simulink model "Hexacopter_2"  (R2017b)
settings: Solver=FixedStepAuto  StartTime=0.0  StopTime=50  FixedStep=0.0001  RelTol=1e-3
values from neighbouring files (symbols this model uses):
  b = 1.14 * 10^(-7)    (= 1.14e-07)    [hexa_parameters.m]
  dPhi_d = 0.0    (= 0)    [hexa_parameters.m]
  dPsi_d = 0.0    (= 0)    [hexa_parameters.m]
  dTheta_d = 0.0    (= 0)    [hexa_parameters.m]
  dx_0 = 0.0    (= 0)    [hexa_parameters.m]
  dy_0 = 0.0    (= 0)    [hexa_parameters.m]
  dz_0 = 0.0    (= 0)    [hexa_parameters.m]
  g = 9.81    [hexa_parameters.m]
  Ir = 3.36 * 10^(-5)    (= 3.36e-05)    [hexa_parameters.m]
  Ixx = 8.80 * 10^(-3)    (= 0.0088)    [hexa_parameters.m]
  Iyy = Ixx    (= 0.0088)    [hexa_parameters.m]
  Izz = 8.80 * 10^(-3)    (= 0.0088)    [hexa_parameters.m]
  k = 2.98 * 10^(-6)    (= 2.98e-06)    [hexa_parameters.m]
  Kphi_d = 0.01    [hexa_parameters.m]
  Kphi_p = 0.01    [hexa_parameters.m]
  Kpsi_d = 0.01    [hexa_parameters.m]
  Kpsi_p = 0.01    [hexa_parameters.m]
  Ktheta_d = 0.01    [hexa_parameters.m]
  Ktheta_p = 0.01    [hexa_parameters.m]
  Kz = 0.1    [hexa_parameters.m]
  Kzd = 1    [hexa_parameters.m]
  l = 1.0    (= 1)    [hexa_parameters.m]
  m = 0.468    [hexa_parameters.m]
  omega = 0.33    [hexa_parameters.m]
  p0 = 0.0    (= 0)    [hexa_parameters.m]
  Phi_d = 0.0    (= 0)    [hexa_parameters.m]
  Psi_d = 0.0    (= 0)    [hexa_parameters.m]
  q0 = 0.0    (= 0)    [hexa_parameters.m]
  q_0 = normalizer_quater(q_0)    [hexa_parameters.m]
  r0 = 0.0    (= 0)    [hexa_parameters.m]
  Theta_d = 0.0    (= 0)    [hexa_parameters.m]
  x_0 = 0.0    (= 0)    [hexa_parameters.m]
  y_0 = 0.0    (= 0)    [hexa_parameters.m]
  z_0 = 1.0    (= 1)    [hexa_parameters.m]
settings Model: Creator=Marco  LastModifiedBy=Marco
settings CodeAppCC: StateflowObjectComments=on

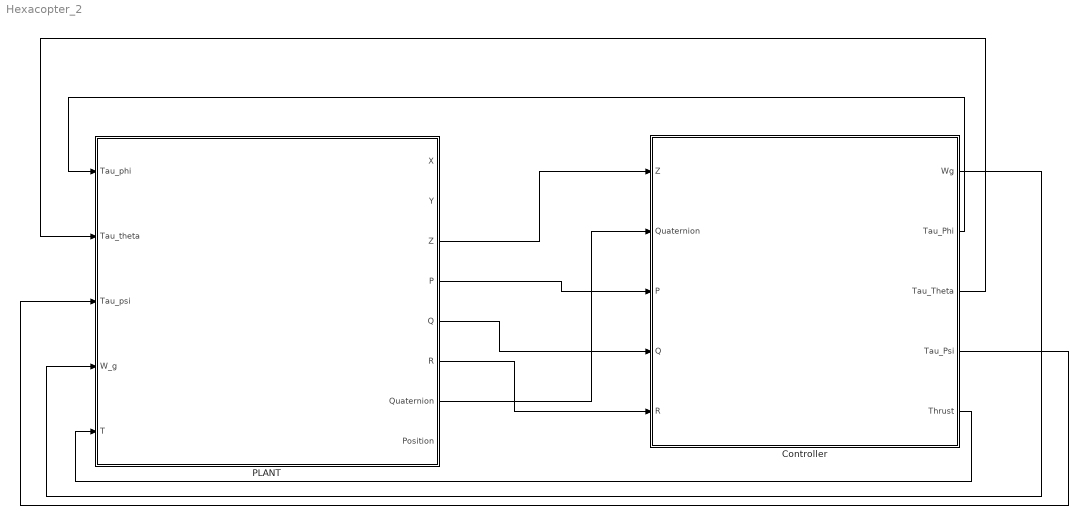
== system Hexacopter_2 ==
  Controller : Subsystem
  PLANT : Subsystem
  wires:
  PLANT/3(Z) -> Controller/1(Z)
  PLANT/7(Quaternion) -> Controller/2(Quaternion)
  PLANT/4(P) -> Controller/3(P)
  PLANT/5(Q) -> Controller/4(Q)
  PLANT/6(R) -> Controller/5(R)
  Controller/1(Wg) -> PLANT/4(W_g)
  Controller/2(Tau_Phi) -> PLANT/1(Tau_phi)
  Controller/3(Tau_Theta) -> PLANT/2(Tau_theta)
  Controller/4(Tau_Psi) -> PLANT/3(Tau_psi)
  Controller/5(Thrust) -> PLANT/5(T)

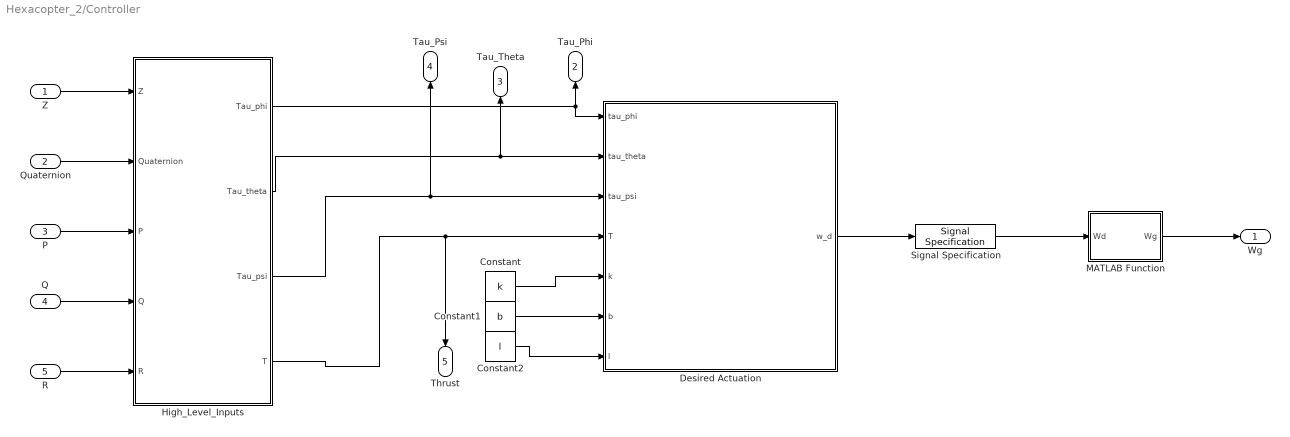
== system Hexacopter_2/Controller ==
  Z : Inport
  Quaternion : Inport  Port=2
  P : Inport  Port=3
  Q : Inport  Port=4
  R : Inport  Port=5
  Constant : Constant  Value=k
  Constant1 : Constant  Value=b
  Constant2 : Constant  Value=l
  Desired Actuation : MATLAB Function  TreatAsAtomicUnit=on
  High_Level_Inputs : Subsystem
  MATLAB Function : MATLAB Function  TreatAsAtomicUnit=on
  Signal Specification : SignalSpecification  Dimensions=[1,6]
  Wg : Outport
  Tau_Phi : Outport  Port=2
  Tau_Theta : Outport  Port=3
  Tau_Psi : Outport  Port=4
  Thrust : Outport  Port=5
  wires:
  High_Level_Inputs/4(T) -> Thrust/1, Desired Actuation/4(T)
  Z/1 -> High_Level_Inputs/1(Z)
  Quaternion/1 -> High_Level_Inputs/2(Quaternion)
  Constant2/1 -> Desired Actuation/7(l)
  Constant1/1 -> Desired Actuation/6(b)
  Constant/1 -> Desired Actuation/5(k)
  MATLAB Function/1(Wg) -> Wg/1
  High_Level_Inputs/1(Tau_phi) -> Desired Actuation/1(tau_phi), Tau_Phi/1
  High_Level_Inputs/2(Tau_theta) -> Tau_Theta/1, Desired Actuation/2(tau_theta)
  High_Level_Inputs/3(Tau_psi) -> Tau_Psi/1, Desired Actuation/3(tau_psi)
  P/1 -> High_Level_Inputs/3(P)
  Q/1 -> High_Level_Inputs/4(Q)
  R/1 -> High_Level_Inputs/5(R)
  Desired Actuation/1(w_d) -> Signal Specification/1
  Signal Specification/1 -> MATLAB Function/1(Wd)

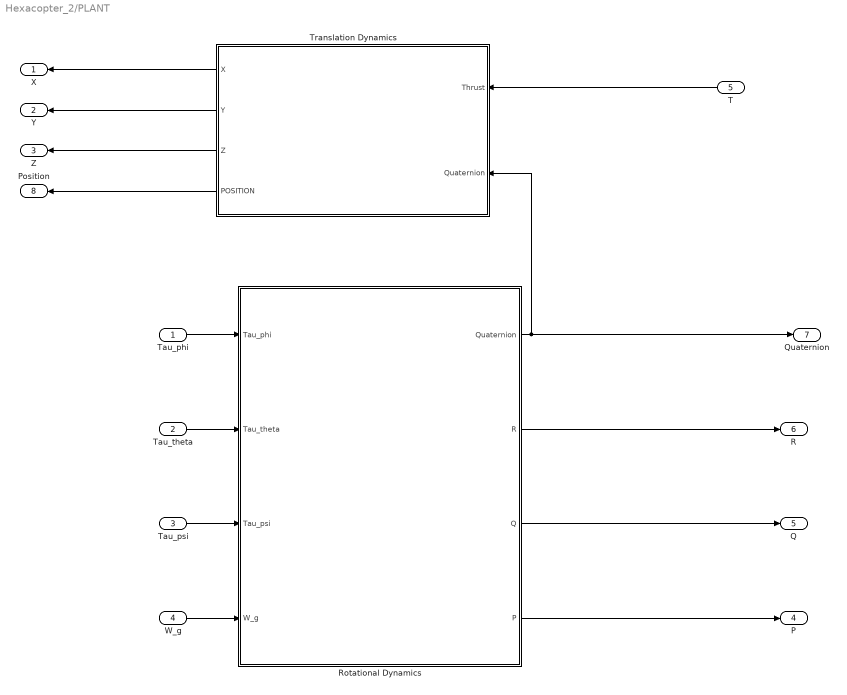
== system Hexacopter_2/PLANT ==
  Tau_phi : Inport
  Tau_theta : Inport  Port=2
  Tau_psi : Inport  Port=3
  W_g : Inport  Port=4
  T : Inport  Port=5
  Rotational Dynamics : Subsystem
  Translation Dynamics : Subsystem
  X : Outport
  Y : Outport  Port=2
  Z : Outport  Port=3
  P : Outport  Port=4
  Q : Outport  Port=5
  R : Outport  Port=6
  Quaternion : Outport  Port=7
  Position : Outport  Port=8
  wires:
  W_g/1 -> Rotational Dynamics/4(W_g)
  Tau_theta/1 -> Rotational Dynamics/2(Tau_theta)
  Tau_phi/1 -> Rotational Dynamics/1(Tau_phi)
  Tau_psi/1 -> Rotational Dynamics/3(Tau_psi)
  T/1 -> Translation Dynamics/1(Thrust)
  Rotational Dynamics/2(R) -> R/1
  Rotational Dynamics/3(Q) -> Q/1
  Rotational Dynamics/4(P) -> P/1
  Translation Dynamics/1(X) -> X/1
  Translation Dynamics/2(Y) -> Y/1
  Translation Dynamics/3(Z) -> Z/1
  Rotational Dynamics/1(Quaternion) -> Translation Dynamics/2(Quaternion), Quaternion/1
  Translation Dynamics/4(POSITION) -> Position/1

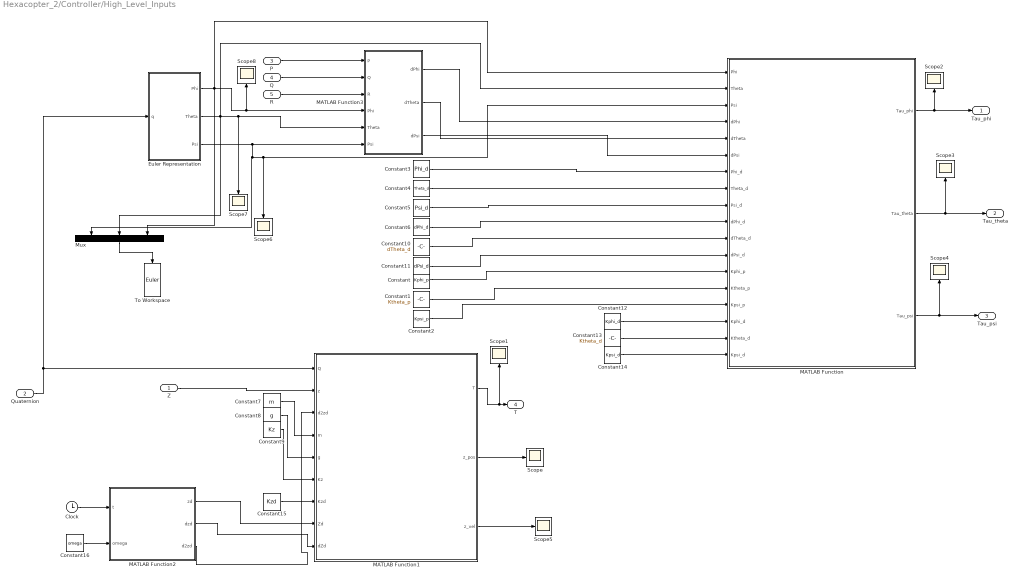
== system Hexacopter_2/Controller/High_Level_Inputs ==
  Z : Inport
  Quaternion : Inport  Port=2
  P : Inport  Port=3
  Q : Inport  Port=4
  R : Inport  Port=5
  Clock : Clock
  Constant : Constant  Value=Kphi_p
  Constant1 : Constant  Value=Ktheta_p
  Constant10 : Constant  Value=dTheta_d
  Constant11 : Constant  Value=dPsi_d
  Constant12 : Constant  Value=Kphi_d
  Constant13 : Constant  Value=Ktheta_d
  Constant14 : Constant  Value=Kpsi_d
  Constant15 : Constant  Value=Kzd
  Constant16 : Constant  Value=omega
  Constant2 : Constant  Value=Kpsi_p
  Constant3 : Constant  Value=Phi_d
  Constant4 : Constant  Value=Theta_d
  Constant5 : Constant  Value=Psi_d
  Constant6 : Constant  Value=dPhi_d
  Constant7 : Constant  Value=m
  Constant8 : Constant  Value=g
  Constant9 : Constant  Value=Kz
  Euler Representation : MATLAB Function  TreatAsAtomicUnit=on
  MATLAB Function : MATLAB Function  TreatAsAtomicUnit=on
  MATLAB Function1 : MATLAB Function  TreatAsAtomicUnit=on
  MATLAB Function2 : MATLAB Function  TreatAsAtomicUnit=on
  MATLAB Function3 : MATLAB Function  TreatAsAtomicUnit=on
  Mux : Mux  Inputs=3
  Scope{,1..8} (9 alike) : Scope
  To Workspace : ToWorkspace  VariableName=Euler  SampleTime=-1
  Tau_phi : Outport
  Tau_theta : Outport  Port=2
  Tau_psi : Outport  Port=3
  T : Outport  Port=4
  wires:
  MATLAB Function1/1(T) -> Scope1/1, T/1
  Z/1 -> MATLAB Function1/2(z)
  Quaternion/1 -> Euler Representation/1(q), MATLAB Function1/1(Q)
  Constant/1 -> MATLAB Function/13(Kphi_p)
  Constant1/1 -> MATLAB Function/14(Ktheta_p)
  Constant2/1 -> MATLAB Function/15(Kpsi_p)
  Euler Representation/1(Phi) -> Mux/3, MATLAB Function/1(Phi), Scope8/1, MATLAB Function3/4(Phi)
  Euler Representation/2(Theta) -> Mux/2, MATLAB Function/2(Theta), Scope7/1, MATLAB Function3/5(Theta)
  Euler Representation/3(Psi) -> Scope6/1, MATLAB Function/3(Psi), Mux/1, MATLAB Function3/6(Psi)
  Constant3/1 -> MATLAB Function/7(Phi_d)
  Constant4/1 -> MATLAB Function/8(Theta_d)
  Constant5/1 -> MATLAB Function/9(Psi_d)
  Constant7/1 -> MATLAB Function1/4(m)
  Constant8/1 -> MATLAB Function1/5(g)
  Constant9/1 -> MATLAB Function1/6(Kz)
  MATLAB Function2/1(zd) -> MATLAB Function1/8(Zd)
  MATLAB Function2/3(d2zd) -> MATLAB Function1/3(d2zd)
  Clock/1 -> MATLAB Function2/1(t)
  P/1 -> MATLAB Function3/1(P)
  Q/1 -> MATLAB Function3/2(Q)
  R/1 -> MATLAB Function3/3(R)
  Constant6/1 -> MATLAB Function/10(dPhi_d)
  Constant10/1 -> MATLAB Function/11(dTheta_d)
  Constant11/1 -> MATLAB Function/12(dPsi_d)
  MATLAB Function3/1(dPhi) -> MATLAB Function/4(dPhi)
  MATLAB Function3/2(dTheta) -> MATLAB Function/5(dTheta)
  MATLAB Function3/3(dPsi) -> MATLAB Function/6(dPsi)
  Constant12/1 -> MATLAB Function/16(Kphi_d)
  Constant13/1 -> MATLAB Function/17(Ktheta_d)
  Constant14/1 -> MATLAB Function/18(Kpsi_d)
  MATLAB Function/1(Tau_phi) -> Scope2/1, Tau_phi/1
  MATLAB Function/2(Tau_theta) -> Scope3/1, Tau_theta/1
  MATLAB Function/3(Tau_psi) -> Scope4/1, Tau_psi/1
  MATLAB Function1/2(z_pos) -> Scope/1
  MATLAB Function2/2(dzd) -> MATLAB Function1/9(dZd)
  Constant15/1 -> MATLAB Function1/7(Kzd)
  MATLAB Function1/3(z_vel) -> Scope5/1
  Constant16/1 -> MATLAB Function2/2(omega)
  Mux/1 -> To Workspace/1

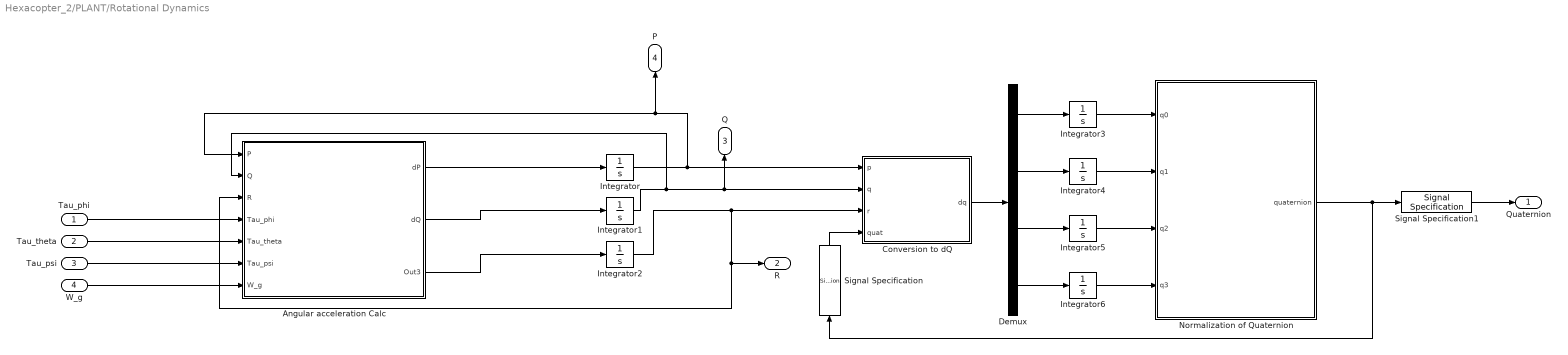
== system Hexacopter_2/PLANT/Rotational Dynamics ==
  Tau_phi : Inport
  Tau_theta : Inport  Port=2
  Tau_psi : Inport  Port=3
  W_g : Inport  Port=4
  " Normalization of Quaternion" : MATLAB Function  TreatAsAtomicUnit=on
  Angular acceleration Calc : Subsystem
  Conversion to dQ : MATLAB Function  TreatAsAtomicUnit=on
  Demux : Demux
  Integrator : Integrator  InitialCondition=p0
  Integrator1 : Integrator  InitialCondition=q0
  Integrator2 : Integrator  InitialCondition=r0
  Integrator3 : Integrator  InitialCondition=q_0(1)
  Integrator4 : Integrator  InitialCondition=q_0(2)
  Integrator5 : Integrator  InitialCondition=q_0(3)
  Integrator6 : Integrator  InitialCondition=q_0(4)
  Signal Specification : SignalSpecification  Dimensions=[1,4]
  Signal Specification1 : SignalSpecification  Dimensions=[1,4]
  Quaternion : Outport
  R : Outport  Port=2
  Q : Outport  Port=3
  P : Outport  Port=4
  wires:
  Demux/1 -> Integrator3/1
  Demux/3 -> Integrator5/1
  Conversion to dQ/1(dq) -> Demux/1
  Integrator1/1 -> Angular acceleration Calc/2(Q), Q/1, Conversion to dQ/2(q)
  Demux/2 -> Integrator4/1
  Integrator2/1 -> R/1, Angular acceleration Calc/3(R), Conversion to dQ/3(r)
  Demux/4 -> Integrator6/1
  Integrator/1 -> Angular acceleration Calc/1(P), P/1, Conversion to dQ/1(p)
  Integrator3/1 -> " Normalization of Quaternion"/1(q0)
  Integrator4/1 -> " Normalization of Quaternion"/2(q1)
  Integrator5/1 -> " Normalization of Quaternion"/3(q2)
  Integrator6/1 -> " Normalization of Quaternion"/4(q3)
  W_g/1 -> Angular acceleration Calc/7(W_g)
  Tau_psi/1 -> Angular acceleration Calc/6(Tau_psi)
  Tau_theta/1 -> Angular acceleration Calc/5(Tau_theta)
  Tau_phi/1 -> Angular acceleration Calc/4(Tau_phi)
  Angular acceleration Calc/1(dP) -> Integrator/1
  Angular acceleration Calc/2(dQ) -> Integrator1/1
  Angular acceleration Calc/3(Out3) -> Integrator2/1
  " Normalization of Quaternion"/1(quaternion) -> Signal Specification/1, Signal Specification1/1
  Signal Specification/1 -> Conversion to dQ/4(quat)
  Signal Specification1/1 -> Quaternion/1

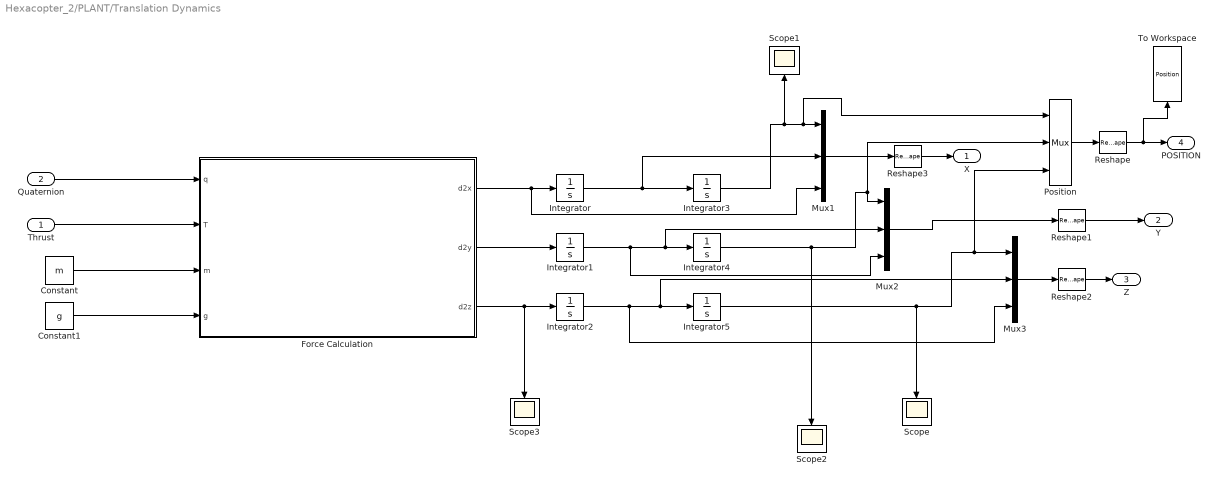
== system Hexacopter_2/PLANT/Translation Dynamics ==
  Thrust : Inport
  Quaternion : Inport  Port=2
  Constant : Constant  Value=m
  Constant1 : Constant  Value=g
  Force Calculation : MATLAB Function  TreatAsAtomicUnit=on
  Integrator : Integrator  InitialCondition=dx_0
  Integrator1 : Integrator  InitialCondition=dy_0
  Integrator2 : Integrator  InitialCondition=dz_0
  Integrator3 : Integrator  InitialCondition=x_0
  Integrator4 : Integrator  InitialCondition=y_0
  Integrator5 : Integrator  InitialCondition=z_0
  Mux1 : Mux  Inputs=3
  Mux2 : Mux  Inputs=3
  Mux3 : Mux  Inputs=3
  Position : Mux  Inputs=3
  Reshape{,1..3} (4 alike) : Reshape  OutputDimensionality=Customize  OutputDimensions=[1,3]
  Scope{,1..3} (4 alike) : Scope
  To Workspace : ToWorkspace  VariableName=Position  SampleTime=-1
  X : Outport
  Y : Outport  Port=2
  Z : Outport  Port=3
  POSITION : Outport  Port=4
  wires:
  Integrator1/1 -> Mux2/3, Mux2/2, Integrator4/1
  Force Calculation/2(d2y) -> Integrator1/1
  Force Calculation/1(d2x) -> Mux1/3, Integrator/1
  Integrator2/1 -> Mux3/3, Mux3/2, Integrator5/1
  Integrator/1 -> Mux1/2, Integrator3/1
  Force Calculation/3(d2z) -> Scope3/1, Integrator2/1
  Mux1/1 -> Reshape3/1
  Mux2/1 -> Reshape1/1
  Mux3/1 -> Reshape2/1
  Integrator3/1 -> Scope1/1, Position/1, Mux1/1
  Integrator4/1 -> Scope2/1, Position/2, Mux2/1
  Integrator5/1 -> Scope/1, Position/3, Mux3/1
  Position/1 -> Reshape/1
  Constant1/1 -> Force Calculation/4(g)
  Quaternion/1 -> Force Calculation/1(q)
  Thrust/1 -> Force Calculation/2(T)
  Constant/1 -> Force Calculation/3(m)
  Reshape/1 -> To Workspace/1, POSITION/1
  Reshape1/1 -> Y/1
  Reshape2/1 -> Z/1
  Reshape3/1 -> X/1

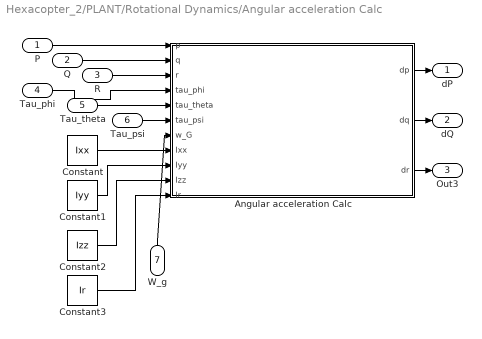
== system Hexacopter_2/PLANT/Rotational Dynamics/Angular acceleration Calc ==
  P : Inport
  Q : Inport  Port=2
  R : Inport  Port=3
  Tau_phi : Inport  Port=4
  Tau_theta : Inport  Port=5
  Tau_psi : Inport  Port=6
  W_g : Inport  Port=7
  Angular acceleration Calc : MATLAB Function  TreatAsAtomicUnit=on
  Constant : Constant  Value=Ixx
  Constant1 : Constant  Value=Iyy
  Constant2 : Constant  Value=Izz
  Constant3 : Constant  Value=Ir
  dP : Outport
  dQ : Outport  Port=2
  Out3 : Outport  Port=3
  wires:
  Q/1 -> Angular acceleration Calc/2(q)
  P/1 -> Angular acceleration Calc/1(p)
  Constant2/1 -> Angular acceleration Calc/10(Izz)
  Constant3/1 -> Angular acceleration Calc/11(Ir)
  Angular acceleration Calc/3(dr) -> Out3/1
  Tau_phi/1 -> Angular acceleration Calc/4(tau_phi)
  Tau_theta/1 -> Angular acceleration Calc/5(tau_theta)
  W_g/1 -> Angular acceleration Calc/7(w_G)
  Tau_psi/1 -> Angular acceleration Calc/6(tau_psi)
  Angular acceleration Calc/1(dp) -> dP/1
  R/1 -> Angular acceleration Calc/3(r)
  Angular acceleration Calc/2(dq) -> dQ/1
  Constant1/1 -> Angular acceleration Calc/9(Iyy)
  Constant/1 -> Angular acceleration Calc/8(Ixx)

== matlab function Hexacopter_2/PLANT/Translation Dynamics/Force Calculation ==
  data: d2x output; d2y output; q input; d2z output; T input; m input; g input
function [d2x,d2y,d2z] = Force_Cal(q,T,m,g)
    d2x = (T/ m) * 2 * (q(1)*q(3) + q(2)*q(4));
    d2y = (T / m) * 2 * (q(3)*q(4) + q(1)*q(2));
    d2z = -g + (T/m) * (q(1)^(2) - q(2)^(2) - q(3)^(2) - q(4)^(2));

== matlab function Hexacopter_2/PLANT/Rotational Dynamics/Angular acceleration Calc/Angular acceleration Calc ==
  data: dp output; p input; q input; r input; tau_phi input; tau_theta input; tau_psi input; w_G input; dq output; dr output; Ixx input; Iyy input; Izz input; Ir input
function [dp,dq,dr] = Angular_Acceleration(p,q,r,tau_phi,tau_theta,tau_psi,w_G,Ixx,Iyy,Izz,Ir)
    dp = ((Iyy-Izz)*q*r - Ir*q*w_G + tau_phi)*(1/Ixx);
    dq = ((Izz-Ixx)*p*r + Ir*p*w_G + tau_theta)*(1/Iyy);
    dr = ((Ixx-Iyy)*p*q +tau_psi)*(1/Izz);

== matlab function Hexacopter_2/PLANT/Rotational Dynamics/Conversion to dQ ==
  data: p input; dq output; q input; r input; quat input
function dq = Conversion_p_dq(p,q,r,quat)
    dq = zeros(1,4);
    dq(1,1) = 0.5 * (-quat(1,2)*p - quat(1,3)*q + quat(1,4)*r);
    dq(1,2) = 0.5 * (quat(1,1)*p - quat(1,4)*q + quat(1,3)*r);
    dq(1,3) = 0.5 * (quat(1,4)*p + quat(1,1)*q - quat(1,2)*r);
    dq(1,4) = 0.5 * (-quat(1,3)*p + quat(1,2)+q + quat(1,1)*r);

== matlab function Hexacopter_2/PLANT/Rotational Dynamics/ Normalization of Quaternion ==
  data: q0 input; quaternion output; q1 input; q2 input; q3 input
function quaternion = quaternioNormalizer(q0,q1,q2,q3)
    quaternion = ones(1,4);
    qtot = sqrt(q0^2+q1^2+q2^2+q3^2);
    norm = 1 / qtot;
    q0 = q0 * norm;
    q1 = q1 * norm;
    q2 = q2 * norm;
    q3 = q3 * norm;
    quaternion = [q0,q1,q2,q3];

== matlab function Hexacopter_2/Controller/High_Level_Inputs/MATLAB Function ==
  data: Phi input; Tau_phi output; Theta input; Psi input; dPhi input; dTheta input; dPsi input; Phi_d input; Theta_d input; Psi_d input; dPhi_d input; dTheta_d input; dPsi_d input; Tau_theta output; Tau_psi output; Kphi_p input; Ktheta_p input; Kpsi_p input; Kphi_d input; Ktheta_d input; Kpsi_d input
function [Tau_phi,Tau_theta,Tau_psi] = Torques(Phi,Theta,Psi,dPhi,dTheta,dPsi,Phi_d,Theta_d,Psi_d,dPhi_d,dTheta_d,dPsi_d,Kphi_p,Ktheta_p,Kpsi_p,Kphi_d,Ktheta_d,Kpsi_d)
Tau_phi = Kphi_p * (Phi_d - Phi) + Kphi_d * (dPhi_d - dPhi);
Tau_theta = Ktheta_p * (Theta_d - Theta) + Ktheta_d * (dTheta_d - dTheta);
Tau_psi = Kpsi_p * (Psi_d - Psi) + Kpsi_d * (dPsi_d - dPsi);

== matlab function Hexacopter_2/Controller/High_Level_Inputs/MATLAB Function1 ==
  data: Q input; T output; z input; d2zd input; m input; g input; Kz input; Kzd input; Zd input; z_pos output; dZd input; z_vel output
function [T,z_pos,z_vel] = Thrust(Q,z,d2zd,m,g,Kz,Kzd,Zd,dZd)

T = m * (d2zd + Kz * (Zd - z(1)) + Kzd * (dZd - z(2)) + g) / (Q(1)^2 - Q(2)^2 - Q(3)^2 + Q(4)^2);
z_pos = z(1);
z_vel = z(2);

== matlab function Hexacopter_2/Controller/MATLAB Function ==
  data: Wd input; Wg output
function Wg = Wg_calculator(Wd)
Wg = -Wd(1) + Wd(2) - Wd(3) + Wd(4) - Wd(5) + Wd(6);

== matlab function Hexacopter_2/Controller/High_Level_Inputs/MATLAB Function2 ==
  data: t input; zd output; dzd output; d2zd output; omega input
function [zd,dzd,d2zd] = Planner(t,omega)

%zd = cos(t*omega);
%dzd = -sin(t*omega);
%d2zd = -cos(t*omega);
zd = 0.0;
dzd = 0.0;
d2zd = 0.0;

== matlab function Hexacopter_2/Controller/High_Level_Inputs/MATLAB Function3 ==
  data: P input; dPhi output; Q input; R input; Phi input; Theta input; Psi input; dTheta output; dPsi output
function [dPhi,dTheta,dPsi] = dEuler(P,Q,R,Phi,Theta,Psi)

dPhi = P + sin(Phi) * tan(Theta) * Q + cos(Phi) * tan(Theta) * R;
dTheta = cos(Phi) * Q - sin(Phi) * R;
dPsi = sec(Theta) * sin(Phi) * Q + cos(Phi) * sec(Theta) * R;

== matlab function Hexacopter_2/Controller/Desired Actuation ==
  data: tau_phi input; tau_theta input; tau_psi input; T input; w_d output; k input; b input; l input
function w_d  = desiredActuation(tau_phi,tau_theta,tau_psi,T,k,b,l)
    w_d = ones(1,6);
    w_d(1,1) = sqrt(T/(6*k) - 2*tau_theta/(5*k*l) - tau_psi/(10*b));
    w_d(1,2) = sqrt(T/(6*k) + tau_phi/(3*k*l) - tau_theta/(5*k*l) + tau_psi/(5*b));
    w_d(1,3) = sqrt(T/(6*k) + tau_phi/(3*k*l) + tau_theta/(5*k*l) - tau_psi/(5*b));
    w_d(1,4) = sqrt(T/(6*k) + 2*tau_theta/(5*k*l) + tau_psi/(10*b));
    w_d(1,5) = sqrt(T/(6*k) - tau_phi/(3*k*l) + tau_theta/(5*k*l) - tau_psi/(5*b));
    w_d(1,6) = sqrt(T/(6*k) - tau_phi/(3*k*l) - tau_theta/(5*k*l) + tau_psi/(5*b));

== matlab function Hexacopter_2/Controller/High_Level_Inputs/Euler Representation ==
  data: q input; Phi output; Theta output; Psi output
function [Phi,Theta,Psi] = quaterToeuler(q)
    Phi   = (atan2(2 *(q(1)*q(2) + q(3)*q(4)),1.0 - 2*(q(2)^2 + q(3)^2)))/(pi);
    Theta = (asin(2*(q(1)*q(3) - q(4)*q(2))))/(pi);
    Psi   = (atan2(2*(q(1)*q(4) + q(2)*q(3)),1.0 - 2*(q(3)^2 + q(4)^2)))/(pi);
